simulink model "Renewable_Energy"  (R2023b)
settings: Solver=VariableStepAuto  StartTime=0.0  StopTime=10.0  RelTol=1e-3
settings Model: Creator=Everest  LastModifiedBy=Everest

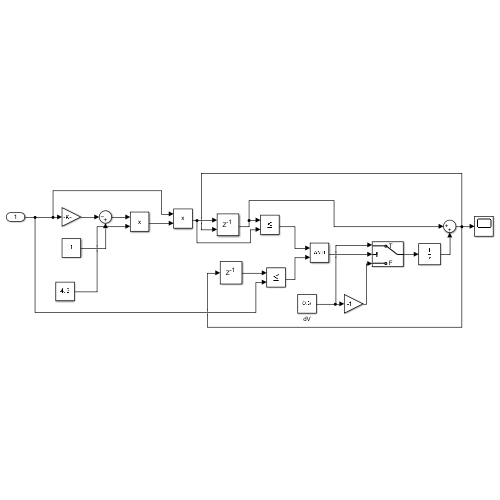
[thumbnail: Simulink's stored preview of the top-level diagram]
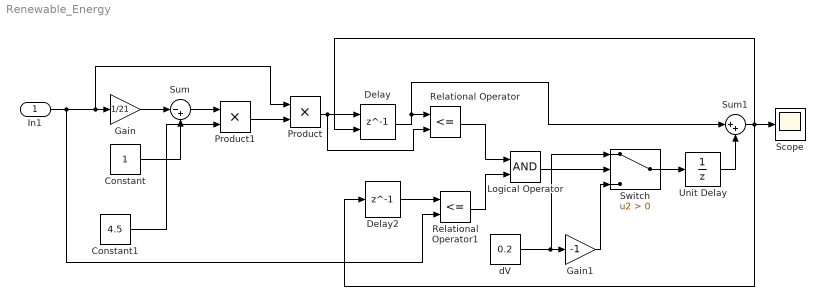
== system Renewable_Energy ==
  In1 : Inport
  Constant : Constant
  Constant1 : Constant  Value=4.5
  Delay : Delay  DelayLength=1  InitialConditionSource=Input port  InitialCondition=5
      settings: InputPortMap=u0,p4
  Delay2 : Delay  DelayLength=1  InitialCondition=5
  Gain : Gain  Gain=1/21
  Gain1 : Gain  Gain=-1
  Logical Operator : Logic  AllPortsSameDT=off  OutDataTypeStr=boolean
  Product : Product
  Product1 : Product
  Relational Operator : RelationalOperator  Operator=<=  OutDataTypeStr=boolean  RndMeth=Simplest  InputSameDT=off
  Relational Operator1 : RelationalOperator  Operator=<=  OutDataTypeStr=boolean  RndMeth=Simplest  InputSameDT=off
  Scope : Scope
  Sum : Sum  Inputs=|-+
  Sum1 : Sum  Inputs=|++
  Switch : Switch  Criteria=u2 > Threshold  SaturateOnIntegerOverflow=off  InputSameDT=off
  Unit Delay : UnitDelay  SampleTime=-1  HasFrameUpgradeWarning=on
  dV : Constant  Value=0.2
  wires:
  In1/1 -> Relational Operator1/2, Product/1, Gain/1
  Gain/1 -> Sum/1
  Constant/1 -> Sum/2
  Sum/1 -> Product1/1
  Constant1/1 -> Product1/2
  Product1/1 -> Product/2
  Delay/1 -> Sum1/1, Relational Operator/1
  Delay2/1 -> Relational Operator1/1
  Relational Operator/1 -> Logical Operator/1
  Relational Operator1/1 -> Logical Operator/2
  Logical Operator/1 -> Switch/2
  dV/1 -> Switch/1, Gain1/1
  Gain1/1 -> Switch/3
  Sum1/1 -> Delay/2, Delay2/1, Scope/1
  Switch/1 -> Unit Delay/1
  Unit Delay/1 -> Sum1/2
  Product/1 -> Delay/1, Relational Operator/2
